simulink model "ControlMultiV1_1_3Robots"  (R2015b)
settings: Solver=ode1  StartTime=0.0  StopTime=inf  FixedStep=0.001  RelTol=1e-3
libraries: simulink x3
settings Model: ExtModeTrigDuration=10000  Creator=ale  LastModifiedBy=anle
settings SolverCC: PositivePriorityOrder=on
settings RTWCC: SystemTargetFile=quarc_linux_duovero.tlc  TemplateMakefile=quarc_linux_duovero_tmf  Description=QUARC Linux DuoVero Target (QBall 2, QBot 2)
settings STFCustomTargetCC: TargetLibSuffix=.a  TargetPreCompLibLocation=C:\PROGRA~3\QUARC\lib\2015b\LINUX_~1\release  GeneratePreprocessorConditionals=Use local settings  CPPClassGenCompliant=off  SystemTargetFile=quarc_linux_duovero.tlc
settings GRTTargetCC: TargetLibSuffix=.a  TargetPreCompLibLocation=C:\PROGRA~3\QUARC\lib\2015b\LINUX_~1\release  ParMdlRefBuildCompliant=off  CompOptLevelCompliant=off  CombineOutputUpdateFcns=off  MatFileLogging=off  CPPClassGenCompliant=off  GRTInterface=on  UseToolchainInfoCompliant=off  ExtMode=on  ExtModeMexFile=quarc_comm  ExtModeMexArgs='-w -d /tmp -uri %u'

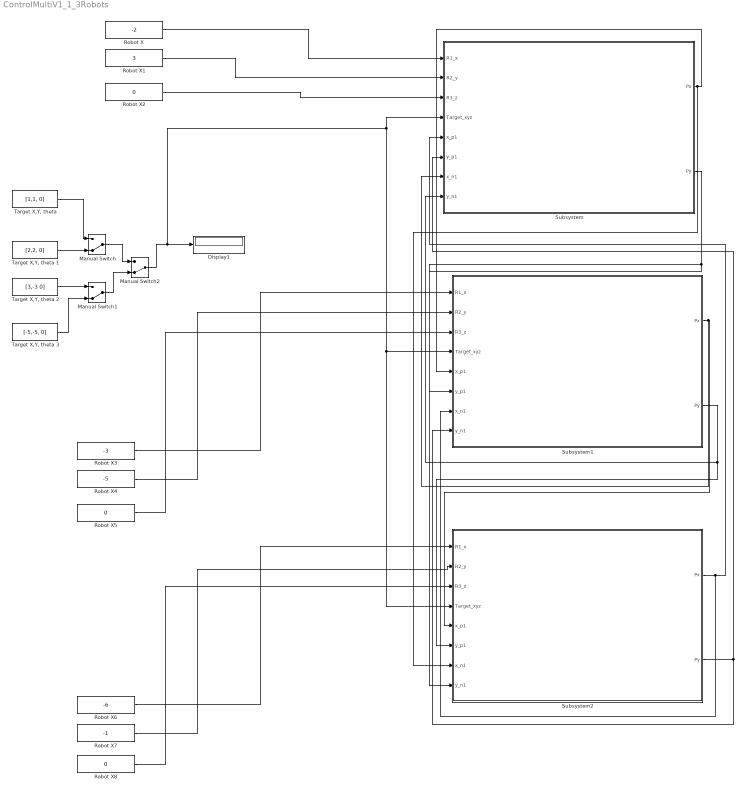
== system ControlMultiV1_1_3Robots ==
  Display1 : Display
  Manual Switch : ManualSwitch  CurrentSetting=0
  Manual Switch1 : ManualSwitch  CurrentSetting=0
  Manual Switch2 : ManualSwitch  CurrentSetting=0
  Robot X : Constant  Value=-2
  Robot X1 : Constant  Value=3
  Robot X2 : Constant  Value=0
  Robot X3 : Constant  Value=-3
  Robot X4 : Constant  Value=-5
  Robot X5 : Constant  Value=0
  Robot X6 : Constant  Value=-6
  Robot X7 : Constant  Value=-1
  Robot X8 : Constant  Value=0
  Subsystem : Subsystem
  Subsystem1 : Subsystem
  Subsystem2 : Subsystem
  "Target X,Y, theta " : Constant  Value=[1,1, 0]
  "Target X,Y, theta 1" : Constant  Value=[2,2, 0]
  "Target X,Y, theta 2" : Constant  Value=[3,-3 0]
  "Target X,Y, theta 3" : Constant  Value=[-5,-5, 0]
  wires:
  Manual Switch2/1 -> Subsystem2/4(Target_xyz), Subsystem1/4(Target_xyz), Subsystem/4(Target_xyz), Display1/1
  "Target X,Y, theta "/1 -> Manual Switch/1
  "Target X,Y, theta 1"/1 -> Manual Switch/2
  Manual Switch/1 -> Manual Switch2/1
  Manual Switch1/1 -> Manual Switch2/2
  "Target X,Y, theta 2"/1 -> Manual Switch1/1
  "Target X,Y, theta 3"/1 -> Manual Switch1/2
  Robot X/1 -> Subsystem/1(R1_x)
  Robot X1/1 -> Subsystem/2(R2_y)
  Robot X2/1 -> Subsystem/3(R3_z)
  Robot X3/1 -> Subsystem1/1(R1_x)
  Robot X4/1 -> Subsystem1/2(R2_y)
  Robot X5/1 -> Subsystem1/3(R3_z)
  Robot X6/1 -> Subsystem2/1(R1_x)
  Robot X7/1 -> Subsystem2/2(R2_y)
  Robot X8/1 -> Subsystem2/3(R3_z)
  Subsystem/1(Px) -> Subsystem2/7(x_n1), Subsystem1/5(x_p1)
  Subsystem/2(Py) -> Subsystem2/8(y_n1), Subsystem1/6(y_p1)
  Subsystem1/1(Px) -> Subsystem/7(x_n1), Subsystem2/5(x_p1)
  Subsystem1/2(Py) -> Subsystem/8(y_n1), Subsystem2/6(y_p1)
  Subsystem2/1(Px) -> Subsystem1/7(x_n1), Subsystem/5(x_p1)
  Subsystem2/2(Py) -> Subsystem/6(y_p1), Subsystem1/8(y_n1)

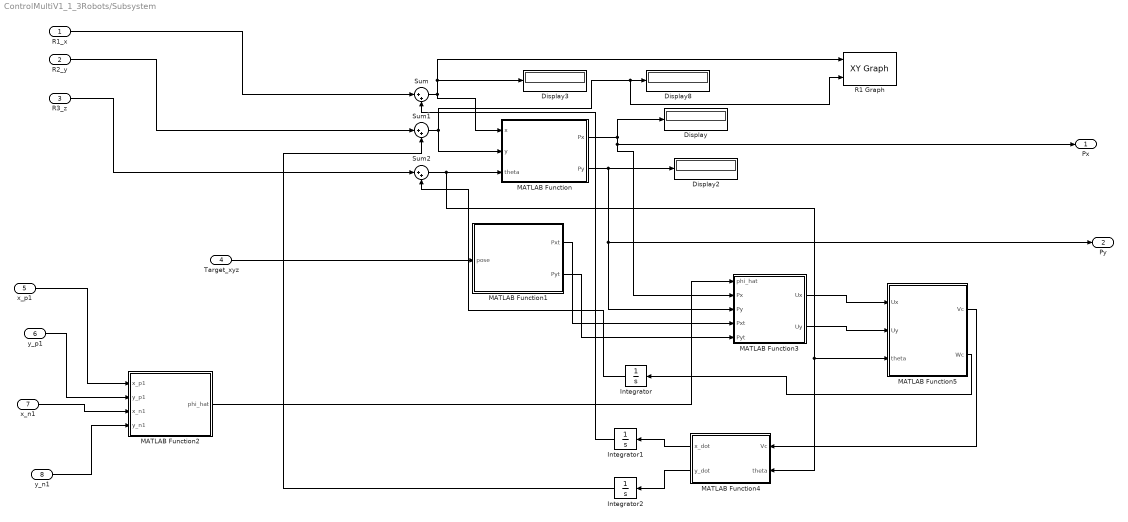
== system ControlMultiV1_1_3Robots/Subsystem ==
  R1_x : Inport
  R2_y : Inport  Port=2
  R3_z : Inport  Port=3
  Target_xyz : Inport  Port=4
  x_p1 : Inport  Port=5
  y_p1 : Inport  Port=6
  x_n1 : Inport  Port=7
  y_n1 : Inport  Port=8
  Display{,2..3,8} (4 alike) : Display
  Integrator : Integrator
  Integrator1 : Integrator
  Integrator2 : Integrator
  MATLAB Function : MATLAB Function  TreatAsAtomicUnit=on
  MATLAB Function1 : MATLAB Function  TreatAsAtomicUnit=on
  MATLAB Function2 : MATLAB Function  TreatAsAtomicUnit=on
  MATLAB Function3 : MATLAB Function  TreatAsAtomicUnit=on
  MATLAB Function4 : MATLAB Function  TreatAsAtomicUnit=on
  MATLAB Function5 : MATLAB Function  TreatAsAtomicUnit=on
  R1 Graph : simulink/Sinks/XY Graph  xmin=-20  xmax=20  ymin=-20  ymax=20  st=-1
  Sum : Sum  Inputs=|++
  Sum1 : Sum  Inputs=|++
  Sum2 : Sum  Inputs=|++
  Px : Outport
  Py : Outport  Port=2
  wires:
  MATLAB Function1/1(Pxt) -> MATLAB Function3/4(Pxt)
  MATLAB Function1/2(Pyt) -> MATLAB Function3/5(Pyt)
  MATLAB Function/2(Py) -> Py/1, MATLAB Function3/3(Py), Display2/1
  MATLAB Function/1(Px) -> MATLAB Function3/2(Px), Px/1, Display/1
  Sum2/1 -> MATLAB Function4/2(theta), MATLAB Function5/3(theta), MATLAB Function/3(theta)
  Sum1/1 -> MATLAB Function/2(y), R1 Graph/2, Display8/1
  Sum/1 -> MATLAB Function/1(x), R1 Graph/1, Display3/1
  Target_xyz/1 -> MATLAB Function1/1(pose)
  MATLAB Function3/1(Ux) -> MATLAB Function5/1(Ux)
  MATLAB Function3/2(Uy) -> MATLAB Function5/2(Uy)
  MATLAB Function5/1(Vc) -> MATLAB Function4/1(Vc)
  MATLAB Function5/2(Wc) -> Integrator/1
  Integrator/1 -> Sum2/2
  MATLAB Function4/1(x_dot) -> Integrator1/1
  Integrator1/1 -> Sum/2
  MATLAB Function4/2(y_dot) -> Integrator2/1
  Integrator2/1 -> Sum1/2
  R1_x/1 -> Sum/1
  R2_y/1 -> Sum1/1
  R3_z/1 -> Sum2/1
  MATLAB Function2/1(phi_hat) -> MATLAB Function3/1(phi_hat)
  x_p1/1 -> MATLAB Function2/1(x_p1)
  y_p1/1 -> MATLAB Function2/2(y_p1)
  x_n1/1 -> MATLAB Function2/3(x_n1)
  y_n1/1 -> MATLAB Function2/4(y_n1)

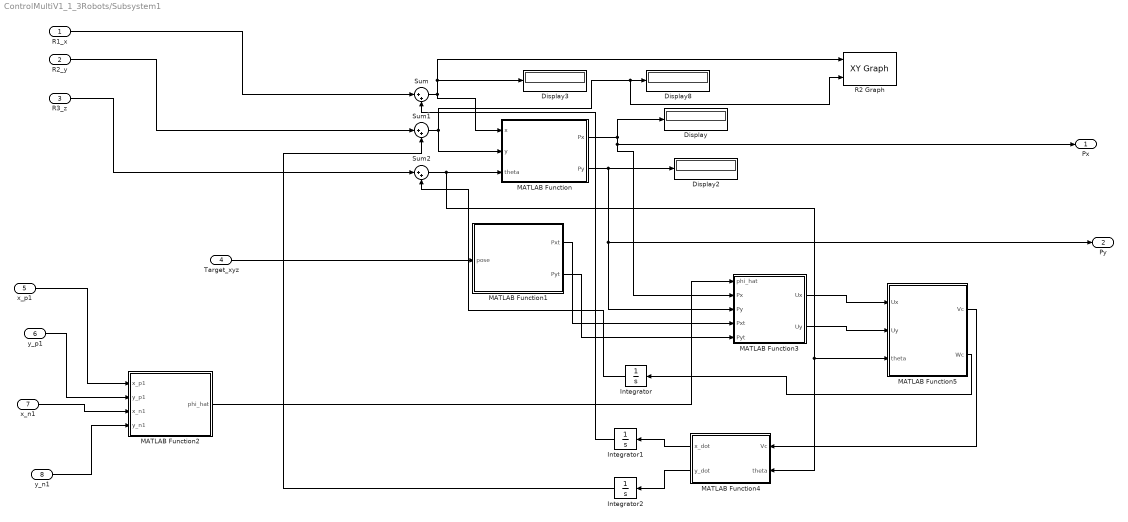
== system ControlMultiV1_1_3Robots/Subsystem1 ==
  R1_x : Inport
  R2_y : Inport  Port=2
  R3_z : Inport  Port=3
  Target_xyz : Inport  Port=4
  x_p1 : Inport  Port=5
  y_p1 : Inport  Port=6
  x_n1 : Inport  Port=7
  y_n1 : Inport  Port=8
  Display{,2..3,8} (4 alike) : Display
  Integrator : Integrator
  Integrator1 : Integrator
  Integrator2 : Integrator
  MATLAB Function : MATLAB Function  TreatAsAtomicUnit=on
  MATLAB Function1 : MATLAB Function  TreatAsAtomicUnit=on
  MATLAB Function2 : MATLAB Function  TreatAsAtomicUnit=on
  MATLAB Function3 : MATLAB Function  TreatAsAtomicUnit=on
  MATLAB Function4 : MATLAB Function  TreatAsAtomicUnit=on
  MATLAB Function5 : MATLAB Function  TreatAsAtomicUnit=on
  R2 Graph : simulink/Sinks/XY Graph  xmin=-20  xmax=20  ymin=-20  ymax=20  st=-1
  Sum : Sum  Inputs=|++
  Sum1 : Sum  Inputs=|++
  Sum2 : Sum  Inputs=|++
  Px : Outport
  Py : Outport  Port=2
  wires:
  MATLAB Function1/1(Pxt) -> MATLAB Function3/4(Pxt)
  MATLAB Function1/2(Pyt) -> MATLAB Function3/5(Pyt)
  MATLAB Function/2(Py) -> Py/1, MATLAB Function3/3(Py), Display2/1
  MATLAB Function/1(Px) -> MATLAB Function3/2(Px), Px/1, Display/1
  Sum2/1 -> MATLAB Function4/2(theta), MATLAB Function5/3(theta), MATLAB Function/3(theta)
  Sum1/1 -> MATLAB Function/2(y), R2 Graph/2, Display8/1
  Sum/1 -> MATLAB Function/1(x), R2 Graph/1, Display3/1
  Target_xyz/1 -> MATLAB Function1/1(pose)
  MATLAB Function3/1(Ux) -> MATLAB Function5/1(Ux)
  MATLAB Function3/2(Uy) -> MATLAB Function5/2(Uy)
  MATLAB Function5/1(Vc) -> MATLAB Function4/1(Vc)
  MATLAB Function5/2(Wc) -> Integrator/1
  Integrator/1 -> Sum2/2
  MATLAB Function4/1(x_dot) -> Integrator1/1
  Integrator1/1 -> Sum/2
  MATLAB Function4/2(y_dot) -> Integrator2/1
  Integrator2/1 -> Sum1/2
  R1_x/1 -> Sum/1
  R2_y/1 -> Sum1/1
  R3_z/1 -> Sum2/1
  MATLAB Function2/1(phi_hat) -> MATLAB Function3/1(phi_hat)
  x_p1/1 -> MATLAB Function2/1(x_p1)
  y_p1/1 -> MATLAB Function2/2(y_p1)
  x_n1/1 -> MATLAB Function2/3(x_n1)
  y_n1/1 -> MATLAB Function2/4(y_n1)

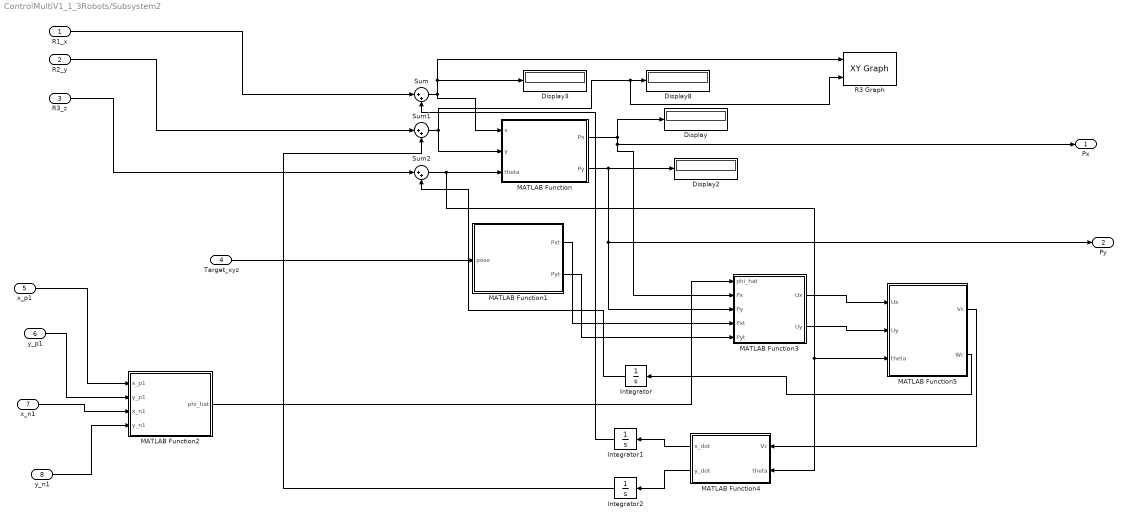
== system ControlMultiV1_1_3Robots/Subsystem2 ==
  R1_x : Inport
  R2_y : Inport  Port=2
  R3_z : Inport  Port=3
  Target_xyz : Inport  Port=4
  x_p1 : Inport  Port=5
  y_p1 : Inport  Port=6
  x_n1 : Inport  Port=7
  y_n1 : Inport  Port=8
  Display{,2..3,8} (4 alike) : Display
  Integrator : Integrator
  Integrator1 : Integrator
  Integrator2 : Integrator
  MATLAB Function : MATLAB Function  TreatAsAtomicUnit=on
  MATLAB Function1 : MATLAB Function  TreatAsAtomicUnit=on
  MATLAB Function2 : MATLAB Function  TreatAsAtomicUnit=on
  MATLAB Function3 : MATLAB Function  TreatAsAtomicUnit=on
  MATLAB Function4 : MATLAB Function  TreatAsAtomicUnit=on
  MATLAB Function5 : MATLAB Function  TreatAsAtomicUnit=on
  R3 Graph : simulink/Sinks/XY Graph  xmin=-20  xmax=20  ymin=-20  ymax=20  st=-1
  Sum : Sum  Inputs=|++
  Sum1 : Sum  Inputs=|++
  Sum2 : Sum  Inputs=|++
  Px : Outport
  Py : Outport  Port=2
  wires:
  MATLAB Function1/1(Pxt) -> MATLAB Function3/4(Pxt)
  MATLAB Function1/2(Pyt) -> MATLAB Function3/5(Pyt)
  MATLAB Function/2(Py) -> Py/1, MATLAB Function3/3(Py), Display2/1
  MATLAB Function/1(Px) -> MATLAB Function3/2(Px), Px/1, Display/1
  Sum2/1 -> MATLAB Function4/2(theta), MATLAB Function5/3(theta), MATLAB Function/3(theta)
  Sum1/1 -> MATLAB Function/2(y), R3 Graph/2, Display8/1
  Sum/1 -> MATLAB Function/1(x), R3 Graph/1, Display3/1
  Target_xyz/1 -> MATLAB Function1/1(pose)
  MATLAB Function3/1(Ux) -> MATLAB Function5/1(Ux)
  MATLAB Function3/2(Uy) -> MATLAB Function5/2(Uy)
  MATLAB Function5/1(Vc) -> MATLAB Function4/1(Vc)
  MATLAB Function5/2(Wc) -> Integrator/1
  Integrator/1 -> Sum2/2
  MATLAB Function4/1(x_dot) -> Integrator1/1
  Integrator1/1 -> Sum/2
  MATLAB Function4/2(y_dot) -> Integrator2/1
  Integrator2/1 -> Sum1/2
  R1_x/1 -> Sum/1
  R2_y/1 -> Sum1/1
  R3_z/1 -> Sum2/1
  MATLAB Function2/1(phi_hat) -> MATLAB Function3/1(phi_hat)
  x_p1/1 -> MATLAB Function2/1(x_p1)
  y_p1/1 -> MATLAB Function2/2(y_p1)
  x_n1/1 -> MATLAB Function2/3(x_n1)
  y_n1/1 -> MATLAB Function2/4(y_n1)

== matlab function ControlMultiV1_1_3Robots/Subsystem1/MATLAB Function ==
  data: x input; Px output; Py output; y input; theta input
function [Px,Py] = PxPy_convert(x, y, theta)

l=.0235; %#length between the two wheels in meters
%R=.0175; %#R or signed distance from ICC (Instanteous center of curvature) in meters
Px= x+l*cos(theta)
Py = y+l*sin(theta)

%#codegen

== matlab function ControlMultiV1_1_3Robots/Subsystem1/MATLAB Function1 ==
  data: pose input; Pxt output; Pyt output
function [Pxt,Pyt] = PxtPyt_convert(pose)
x=pose(1);
y=pose(2);
theta=pose(2);
l=.0235; %#length between the two wheels in meters
%R=.0175; %#R or signed distance from ICC (Instanteous center of curvature) in meters
Pxt= x+l*cos(theta)
Pyt = y+l*sin(theta)

%#codegen

== matlab function ControlMultiV1_1_3Robots/Subsystem1/MATLAB Function2 ==
  data: x_p1 input; phi_hat output; y_p1 input; x_n1 input; y_n1 input
function phi_hat  = rho_phi_convert(x_p1,y_p1,x_n1,y_n1)
%x_p1,y_p1,x_n1,y_n1 are for phi_i+1, phi_i-1

[phi_p1, rho] = cart2pol((x_p1),(y_p1))

[phi_n1, rho] = cart2pol((x_n1),(y_n1))

phi_hat = (phi_p1+phi_n1+2*pi)/2

== matlab function ControlMultiV1_1_3Robots/Subsystem1/MATLAB Function3 ==
  data: phi_hat input; Px input; Ux output; Py input; Pxt input; Pyt input; Uy output
function [Ux, Uy] = UxUy(phi_hat,Px,Py,Pxt,Pyt)
%#codegen
%rho_star=.5;
%omega_star=.5;
 
krho = 0.5;
kphi = 1;
w_d=1;
 
U = [0 0];
rho_size = 1;
phi_size = 1;
[phi, rho] = cart2pol(Px,Py);
[phi_d, rho_d] = cart2pol(Pxt,Pyt);
 
[phi_dif, rho_dif] = cart2pol((Px-Pxt),(Py-Pyt));
 
PxD = Px - Pxt; 
PyD = Py - Pyt;
 
 
 
J_i=[PxD/(sqrt(PxD^2+PyD^2)) PyD/(sqrt(PxD^2+PyD^2)); -PyD/(PxD^2+PyD^2) PxD/(PxD^2+PyD^2)];
 
 
 
 
%J_i=[(Px-Pxt)/phi_dif (Py-Pyt)/phi_dif;...
%    -(Py-Pyt)/((1+((Py-Pyt)/(PD))^2)*(Px-Pxt)^2)  1/((1+((Py-Pyt)/(PD))^2)*(Px-Pxt))];
 
 
 
%J_i=[ (Px-Pxt)/phi (Py-Pyt)/phi_dif;    -(Py-Pyt)/(phi_dif)^2  (Px-Pxt)/(phi_dif)^2 ];
 
rhoi_dot = krho*(rho_size-rho_dif)
phii_dot = w_d + kphi*(phi_hat-phi);
V_i= [rhoi_dot; phii_dot];
Rt = [ 1 0; 0 1];
 
 
U = Rt*(J_i'*V_i);
U = inv(J_i)*V_i; 
Ux = U(1);
Uy = U(2);

== matlab function ControlMultiV1_1_3Robots/Subsystem1/MATLAB Function4 ==
  data: Vc input; x_dot output; theta input; y_dot output
function [x_dot, y_dot] = VcWc2XYdot(Vc, theta)
%#codegen
x_dot = Vc*cos(theta)
y_dot = Vc*sin(theta)

== matlab function ControlMultiV1_1_3Robots/Subsystem1/MATLAB Function5 ==
  data: Ux input; Vc output; Uy input; Wc output; theta input
function [Vc,Wc] = UxUy2VcWc(Ux,Uy, theta)

l=.0235; %#length between the two wheels in meters
kin_inv = inv([cos(theta) -l*sin(theta) ; sin(theta) l*cos(theta)]);
P =  kin_inv*[Ux;Uy];
Vc=P(1);
Wc=P(2);

== matlab function ControlMultiV1_1_3Robots/Subsystem2/MATLAB Function ==
  data: x input; Px output; Py output; y input; theta input
function [Px,Py] = PxPy_convert(x, y, theta)

l=.0235; %#length between the two wheels in meters
%R=.0175; %#R or signed distance from ICC (Instanteous center of curvature) in meters
Px= x+l*cos(theta)
Py = y+l*sin(theta)

%#codegen

== matlab function ControlMultiV1_1_3Robots/Subsystem2/MATLAB Function1 ==
  data: pose input; Pxt output; Pyt output
function [Pxt,Pyt] = PxtPyt_convert(pose)
x=pose(1);
y=pose(2);
theta=pose(2);
l=.0235; %#length between the two wheels in meters
%R=.0175; %#R or signed distance from ICC (Instanteous center of curvature) in meters
Pxt= x+l*cos(theta)
Pyt = y+l*sin(theta)

%#codegen

== matlab function ControlMultiV1_1_3Robots/Subsystem2/MATLAB Function2 ==
  data: x_p1 input; phi_hat output; y_p1 input; x_n1 input; y_n1 input
function phi_hat  = rho_phi_convert(x_p1,y_p1,x_n1,y_n1)
%x_p1,y_p1,x_n1,y_n1 are for phi_i+1, phi_i-1

[phi_p1, rho] = cart2pol((x_p1),(y_p1))

[phi_n1, rho] = cart2pol((x_n1),(y_n1))

phi_hat = (phi_p1+phi_n1+2*pi)/2

== matlab function ControlMultiV1_1_3Robots/Subsystem2/MATLAB Function3 ==
  data: phi_hat input; Px input; Ux output; Py input; Pxt input; Pyt input; Uy output
function [Ux, Uy] = UxUy(phi_hat,Px,Py,Pxt,Pyt)
%#codegen
%rho_star=.5;
%omega_star=.5;
 
krho = 0.5;
kphi = 1;
w_d=1;
 
U = [0 0];
rho_size = 1;
phi_size = 1;
[phi, rho] = cart2pol(Px,Py);
[phi_d, rho_d] = cart2pol(Pxt,Pyt);
 
[phi_dif, rho_dif] = cart2pol((Px-Pxt),(Py-Pyt));
 
PxD = Px - Pxt; 
PyD = Py - Pyt;
 
 
 
J_i=[PxD/(sqrt(PxD^2+PyD^2)) PyD/(sqrt(PxD^2+PyD^2)); -PyD/(PxD^2+PyD^2) PxD/(PxD^2+PyD^2)];
 
 
 
 
%J_i=[(Px-Pxt)/phi_dif (Py-Pyt)/phi_dif;...
%    -(Py-Pyt)/((1+((Py-Pyt)/(PD))^2)*(Px-Pxt)^2)  1/((1+((Py-Pyt)/(PD))^2)*(Px-Pxt))];
 
 
 
%J_i=[ (Px-Pxt)/phi (Py-Pyt)/phi_dif;    -(Py-Pyt)/(phi_dif)^2  (Px-Pxt)/(phi_dif)^2 ];
 
rhoi_dot = krho*(rho_size-rho_dif)
phii_dot = w_d + kphi*(phi_hat-phi);
V_i= [rhoi_dot; phii_dot];
Rt = [ 1 0; 0 1];
 
 
U = Rt*(J_i'*V_i);
U = inv(J_i)*V_i; 
Ux = U(1);
Uy = U(2);

== matlab function ControlMultiV1_1_3Robots/Subsystem2/MATLAB Function4 ==
  data: Vc input; x_dot output; theta input; y_dot output
function [x_dot, y_dot] = VcWc2XYdot(Vc, theta)
%#codegen
x_dot = Vc*cos(theta)
y_dot = Vc*sin(theta)

== matlab function ControlMultiV1_1_3Robots/Subsystem2/MATLAB Function5 ==
  data: Ux input; Vc output; Uy input; Wc output; theta input
function [Vc,Wc] = UxUy2VcWc(Ux,Uy, theta)

l=.0235; %#length between the two wheels in meters
kin_inv = inv([cos(theta) -l*sin(theta) ; sin(theta) l*cos(theta)]);
P =  kin_inv*[Ux;Uy];
Vc=P(1);
Wc=P(2);

== matlab function ControlMultiV1_1_3Robots/Subsystem/MATLAB Function ==
  data: x input; Px output; Py output; y input; theta input
function [Px,Py] = PxPy_convert(x, y, theta)

l=.0235; %#length between the two wheels in meters
%R=.0175; %#R or signed distance from ICC (Instanteous center of curvature) in meters
Px= x+l*cos(theta)
Py = y+l*sin(theta)

%#codegen

== matlab function ControlMultiV1_1_3Robots/Subsystem/MATLAB Function1 ==
  data: pose input; Pxt output; Pyt output
function [Pxt,Pyt] = PxtPyt_convert(pose)
x=pose(1);
y=pose(2);
theta=pose(2);
l=.0235; %#length between the two wheels in meters
%R=.0175; %#R or signed distance from ICC (Instanteous center of curvature) in meters
Pxt= x+l*cos(theta)
Pyt = y+l*sin(theta)

%#codegen

== matlab function ControlMultiV1_1_3Robots/Subsystem/MATLAB Function2 ==
  data: x_p1 input; phi_hat output; y_p1 input; x_n1 input; y_n1 input
function phi_hat  = rho_phi_convert(x_p1,y_p1,x_n1,y_n1)
%x_p1,y_p1,x_n1,y_n1 are for phi_i+1, phi_i-1

[phi_p1, rho] = cart2pol((x_p1),(y_p1))

[phi_n1, rho] = cart2pol((x_n1),(y_n1))

phi_hat = (phi_p1+phi_n1+2*pi)/2

== matlab function ControlMultiV1_1_3Robots/Subsystem/MATLAB Function3 ==
  data: phi_hat input; Px input; Ux output; Py input; Pxt input; Pyt input; Uy output
function [Ux, Uy] = UxUy(phi_hat,Px,Py,Pxt,Pyt)
%#codegen
%rho_star=.5;
%omega_star=.5;
 
krho = 0.5;
kphi = 1;
w_d=1;
 
U = [0 0];
rho_size = 1;
phi_size = 1;
[phi, rho] = cart2pol(Px,Py);
[phi_d, rho_d] = cart2pol(Pxt,Pyt);
 
[phi_dif, rho_dif] = cart2pol((Px-Pxt),(Py-Pyt));
 
PxD = Px - Pxt; 
PyD = Py - Pyt;
 
 
 
J_i=[PxD/(sqrt(PxD^2+PyD^2)) PyD/(sqrt(PxD^2+PyD^2)); -PyD/(PxD^2+PyD^2) PxD/(PxD^2+PyD^2)];
 
 
 
 
%J_i=[(Px-Pxt)/phi_dif (Py-Pyt)/phi_dif;...
%    -(Py-Pyt)/((1+((Py-Pyt)/(PD))^2)*(Px-Pxt)^2)  1/((1+((Py-Pyt)/(PD))^2)*(Px-Pxt))];
 
 
 
%J_i=[ (Px-Pxt)/phi (Py-Pyt)/phi_dif;    -(Py-Pyt)/(phi_dif)^2  (Px-Pxt)/(phi_dif)^2 ];
 
rhoi_dot = krho*(rho_size-rho_dif)
phii_dot = w_d + kphi*(phi_hat-phi);
V_i= [rhoi_dot; phii_dot];
Rt = [ 1 0; 0 1];
 
 
U = Rt*(J_i'*V_i);
U = inv(J_i)*V_i; 
Ux = U(1);
Uy = U(2);

== matlab function ControlMultiV1_1_3Robots/Subsystem/MATLAB Function4 ==
  data: Vc input; x_dot output; theta input; y_dot output
function [x_dot, y_dot] = VcWc2XYdot(Vc, theta)
%#codegen
x_dot = Vc*cos(theta)
y_dot = Vc*sin(theta)

== matlab function ControlMultiV1_1_3Robots/Subsystem/MATLAB Function5 ==
  data: Ux input; Vc output; Uy input; Wc output; theta input
function [Vc,Wc] = UxUy2VcWc(Ux,Uy, theta)

l=.0235; %#length between the two wheels in meters
kin_inv = inv([cos(theta) -l*sin(theta) ; sin(theta) l*cos(theta)]);
P =  kin_inv*[Ux;Uy];
Vc=P(1);
Wc=P(2);
